simulink model "TV_2017old"  (R2016a)
settings: Solver=FixedStepAuto  StartTime=0.0  StopTime=inf  FixedStep=0.001  RelTol=1e-3
PreLoadFcn:
  | TV_2017_parameters
values from neighbouring files (symbols this model uses):
  battery_voltage = single(530)    [HIL_parameters.m]    (also in HIL_parameters_2018.m; TV_2017_parameters.m; TV_2017_parameters_VD.m)
  car_params = Simulink_Car_params    [HIL_parameters.m]    (also in HIL_parameters_2018.m; TV_2017_parameters.m; TV_2017_parameters_VD.m)
  i_Diff = 16    [HIL_parameters.m]    (also in HIL_parameters_2018.m; TV_2017_parameters.m)
  Kp = 1    [HIL_parameters.m]    (also in HIL_parameters_2018.m; TV_2017_parameters.m; TV_2017_parameters_VD.m)
  motor_data = struct    [HIL_parameters.m]    (also in HIL_parameters_2018.m; TV_2017_parameters.m)
  powerLimitControl = Simulink_el    [HIL_parameters.m]    (also in HIL_parameters_2018.m; TV_2017_parameters.m; TV_2017_parameters_VD.m)
  settings = Simulink_Settings    [HIL_parameters.m]    (also in HIL_parameters_2018.m; TV_2017_parameters.m; TV_2017_parameters_VD.m)
  SpdC_BCC = 0    [HIL_parameters.m]    (also in HIL_parameters_2018.m; TV_2017_parameters.m; TV_2017_parameters_VD.m)
  Speed_Neg_sat = -21    [HIL_parameters.m]    (also in HIL_parameters_2018.m; TV_2017_parameters.m; TV_2017_parameters_VD.m)
  Speed_Pos_sat = 21    [HIL_parameters.m]    (also in HIL_parameters_2018.m; TV_2017_parameters.m; TV_2017_parameters_VD.m)
  SteeringAngleFL = [-23.80 -22.65 -21.50 -20.34 -19.18 -18.03 -16.86 -15.70 -14.53 -13.35 -12.18 -10.99 -9.80 -8.61 -7.40 -6.19 -4.97 -3.75 -2.51 -1.26 0 1.27 2.56 3.85 5.17 6.50 7.84 9.21 10.59 12.00 13.42 14.88 16.36 17.87 19.41 20.99 22.61 24.26 25.97 27.73 29.54]    [CarSetupAnalysis2018.m]    (also in HIL_parameters_2018.m; TV_2017_parameters.m; TV_2017_parameters_VD.m = [-24.129 -22.950 -21.772 -20.593 -19.413 -18.232 -17.050 -15)
  SteeringAngleFR = [-29.54 -27.73 -25.97 -24.26 -22.61 -20.99 -19.41 -17.87 -16.36 -14.88 -13.42 -12.00 -10.59 -9.21 -7.84 -6.50 -5.17 -3.85 -2.56 -1.27 0 1.26 2.51 3.75 4.97 6.19 7.40 8.61 9.80 10.99 12.18 13.35 14.53 15.70 16.86 18.03 19.18 20.34 21.50 22.65 23.80]    [CarSetupAnalysis2018.m]    (also in HIL_parameters_2018.m; TV_2017_parameters.m; TV_2017_parameters_VD.m = [-29.3050 -27.5340 -25.8140 -24.1410 -22.5110 -20.9180 -19.3)
  SteeringWhAngle = [-105 -99.75 -94.5 -89.25 -84 -78.75 -73.5 -68.25 -63 -57.75 -52.5 -47.25 -42 -36.75 -31.5 -26.25 -21.0 -15.75 -10.5 -5.25 0.0 5.25 10.50 15.75 21.00 26.25 31.50 36.75 42.00 47.25 52.50 57.75  63.00 68.25 73.50 78.75 84.00 89.25 94.50 99.75 105.00]    [TV_2017_parameters_VD.m]
  Tn_n = 0    [HIL_parameters.m]    (also in HIL_parameters_2018.m; TV_2017_parameters.m; TV_2017_parameters_VD.m)
  tractionControl = Simulink_tc    [HIL_parameters.m]    (also in HIL_parameters_2018.m; IterativeTractionControlTuning.m; TV_2017_parameters.m; TV_2017_parameters_VD.m)
  yawRateControl = Simulink_yawRate    [HIL_parameters.m]    (also in HIL_parameters_2018.m; TV_2017_parameters.m; TV_2017_parameters_VD.m)
undefined symbols (not defined in the file or in its folder): DiscIntNeverNeededParam, magnitude, speedEstimation, TC_Decr_Gas, TC_Derivative, TC_Incr_Gas, TC_On, TC_Relay_Off, TC_Relay_On
libraries: CarMaker4SL x274, simulink_extras x45, simulink x37, dspfdesign x2
(part 9 of 14)

== matlab function TV_2017old/CarMaker/Control_System /Torque allocation 2016/Torque Allocation/TorqueAllocation ==
  data: Ti_lim output Bus: Ti_lim; T_req input; states input; maxMotorTorque input; settings parameter; car_params parameter; Mz_ref input; Ti_max output; Mz_error output; Mz_allocated output; yawRateControl parameter
function [Ti_lim,Ti_max,Mz_error, Mz_allocated]  = torqueAllocation(T_req,states,maxMotorTorque,settings, car_params, Mz_ref,yawRateControl)
%#codegen

%STATES
r = states.r;
negative_torque_limit = yawRateControl.negative_torque_limit;

%PARAMETERS
%mu = states.mu;
mu = settings.mu;
tf = car_params.t_f*2;
tr = car_params.t_r*2;
GR = car_params.GR;
r_eff = car_params.r_eff;
R = [r_eff; r_eff; r_eff; r_eff]';


Fzi = [max(1,states.Fz_FL) max(1,states.Fz_FR) max(1,states.Fz_RL) max(1,states.Fz_RR)]';
switch settings.TV_Method
    case 1
        % Only positive Torque
       alfa_r =  (Fzi(3) + Fzi(4)) / (Fzi(1) + Fzi(2) + Fzi(3) + Fzi(4));
    case 2
        % Can also allocate negative torque
       alfa_r =  (Fzi(3) + Fzi(4)) / (Fzi(1) + Fzi(2) + Fzi(3) + Fzi(4));
       %alfa_r = single(0.5)  test dette for å se om distribusjonen blir
       %lik ev soverestimer friksjonspotensialet
    case 3
        % Static 25 percent to each wheel
        alfa_r = single(0.5);
    case 4
        % Allocation with negative torque, but does not use Fz
        alfa_r = single(0.5); 
    otherwise
        alfa_r = single(0.5);       
end

S = states.wheel_angle;

l1 = car_params.t_f*cos(S);
l2 = car_params.t_f*cos(S);
l3 = car_params.t_r;
l4 = car_params.t_r;
L = [-l1; l2; -l3; l4];



%FIND MAXIMUM ALLOWED MOTOR TORQUE, TIRE/MOTOR
Ti_max          = single(zeros(4,1));
Ti_max_tire     = single(zeros(4,1));

RPM = [states.RPM_FL, states.RPM_FR, states.RPM_RL, states.RPM_RR];
Ti_max_motor = [maxMotorTorque.mmt_FL,maxMotorTorque.mmt_FR,maxMotorTorque.mmt_RL,maxMotorTorque.mmt_RR]; 

%Tire saturation based on mu and Fz
for i=1:4
    Ti_max_tire(i) = Fzi(i)*mu*R(i)/GR;
end

%Find minimum of tire saturation Torque and motor
for i=1:4
    Ti_max(i) = min(Ti_max_tire(i), Ti_max_motor(i));
end
%**********************************************%

T_F = single(zeros(2,1));
T_R = single(zeros(2,1));
sat_F = uint32(0);
sat_R = uint32(0);

if ( T_req >= 0)
    switch settings.TV_Method
        case 1
            % Only positive Torque
            [T_F, sat_F] = allocatePositiveTorque(Ti_max(1), Ti_max(2), T_req, R(1), R(2), (1-alfa_r), Mz_ref, GR, tf);
            [T_R, sat_R] = allocatePositiveTorque(Ti_max(3), Ti_max(4), T_req, R(3), R(4), alfa_r, Mz_ref, GR, tr);
        case 2
            % Can also allocate negative torque
            [T_F, sat_F] = allocateTorque(Ti_max(1), Ti_max(2), T_req, R(1), R(2), (1-alfa_r), Mz_ref, GR, tf, negative_torque_limit);
            [T_R, sat_R] = allocateTorque(Ti_max(3), Ti_max(4), T_req, R(3), R(4), alfa_r, Mz_ref, GR, tr ,negative_torque_limit);
        case 3
            % Static 25 percent to each wheel
            T_F = [0.25*T_req; 0.25*T_req];
            T_R = [0.25*T_req; 0.25*T_req];
        case 4
            % Allocation with negative torque, but does not use Fz
            [T_F, sat_F] = allocateTorque(Ti_max_motor(1), Ti_max_motor(2), T_req, R(1), R(2), (1-alfa_r), Mz_ref, GR, tf, negative_torque_limit);
            [T_R, sat_R] = allocateTorque(Ti_max_motor(3), Ti_max_motor(4), T_req, R(3), R(4), alfa_r, Mz_ref, GR, tr ,negative_torque_limit);
    end
            
    if ( (sat_F == 1) && (sat_R == 1) )
        % Nothing more to do
    elseif ( (sat_F == 1) && (sat_R == 0) )     
         if ( T_F(1) < 0) 
            T_remaining = T_req - (T_F(2));
         elseif (T_F(2) < 0) 
             T_remaining = T_req - (T_F(1));
         else
             T_remaining = T_req - (T_F(1) + T_F(2));
         end
         
         if (yawRateControl.enable == 1)
             Mz_remaining = Mz_ref - (-l1*GR*T_F(1)/R(1) + l2*GR*T_F(2)/R(2));
         else
             Mz_remaining = single(0);
         end 
         
        switch settings.TV_Method
            case 1
                % Only positive Torque
                [T_R sat_R] = allocatePositiveTorque(Ti_max(3), Ti_max(4), T_remaining, R(3), R(4), 1 , Mz_remaining, GR, tr);
            case 2
                % Can also allocate negative torque
                [T_R sat_R] = allocateTorque(Ti_max(3), Ti_max(4), T_remaining, R(3), R(4), 1 , Mz_remaining, GR, tr,negative_torque_limit);
            case 4
                [T_R sat_R] = allocateTorque(Ti_max_motor(3), Ti_max_motor(4), T_remaining, R(3), R(4), 1 , Mz_remaining, GR, tr,negative_torque_limit);
        end 
    elseif ( (sat_F == 0) && (sat_R == 1) )
         if ( T_R(1) < 0) 
            T_remaining = T_req - (T_R(2));
         elseif (T_R(2) < 0) 
             T_remaining = T_req - (T_R(1));
         else
             T_remaining = T_req - (T_R(1) + T_R(2));
         end        
        % For example rear is saturated, and front can still use more torque
        %T_remaining = T_req - (T_R(1) + T_R(2));
        if (yawRateControl.enable == 1)
             Mz_remaining = Mz_ref - (-l3*GR*T_R(1)/R(3) + l4*GR*T_R(2)/R(4));
        else
             Mz_remaining = single(0);
        end 
        %Mz_remaining = Mz_ref*(1-alfa_r);
        switch settings.TV_Method
            case 1
                % Only positive Torque
                 [T_F sat_F] = allocatePositiveTorque(Ti_max(1), Ti_max(2), T_remaining, R(1), R(2), 1 , Mz_remaining, GR, tf);
            case 2
                % Can also allocate negative torque
                [T_F sat_F] = allocateTorque(Ti_max(1), Ti_max(2), T_remaining, R(1), R(2), 1 , Mz_remaining, GR, tf,negative_torque_limit);
            case 4
                [T_F sat_F] = allocateTorque(Ti_max_motor(1), Ti_max_motor(2), T_remaining, R(1), R(2), 1 , Mz_remaining, GR, tf,negative_torque_limit);
        end      
    else
        %both false
        % Nothing to do here either
    end
else
    %REGENERATIVE BRAKE COMMAND ( T_DRIVER_REQ < 0 )
    switch settings.TV_Method
        case 1
            % Only positive Torque
            [T_F, sat_F] = allocateKersTorque(Ti_max(1), Ti_max(2), T_req, R(1), R(2), (1-alfa_r), Mz_ref, GR, tf);
            [T_R, sat_R] = allocateKersTorque(Ti_max(3), Ti_max(4), T_req, R(3), R(4), alfa_r, Mz_ref, GR, tr);
            
        case 2
            % Can also allocate negative torque
            [T_F, sat_F] = allocateKersTorque(Ti_max(1), Ti_max(2), T_req, R(1), R(2), (1-alfa_r), Mz_ref, GR, tf);
            [T_R, sat_R] = allocateKersTorque(Ti_max(3), Ti_max(4), T_req, R(3), R(4), alfa_r, Mz_ref, GR, tr);
        case 3
            % Static 25 percent to each wheel
            T_F = [0.25*T_req; 0.25*T_req];
            T_R = [0.25*T_req; 0.25*T_req];
        case 4
            % Allocation with negative torque, but does not use Fz
            [T_F, sat_F] = allocateKersTorque(Ti_max_motor(1), Ti_max_motor(2), T_req, R(1), R(2), (1-alfa_r), Mz_ref, GR, tf);
            [T_R, sat_R] = allocateKersTorque(Ti_max_motor(3), Ti_max_motor(4), T_req, R(3), R(4), alfa_r, Mz_ref, GR, tr);
    end
    if (sat_F == 1 && sat_R == 1)
        %Nothing more to do
        
    elseif (sat_F == 1 && sat_R == 0)
         T_remaining = T_req - (T_F(1) + T_F(2));
         %Disable Mz_remaining if yaw control disabled?
        if (yawRateControl.enable == 1)
             Mz_remaining = Mz_ref - (-l1*GR*T_F(1)/R(1) + l2*GR*T_F(2)/R(2));
        else
             Mz_remaining = single(0);
        end
        switch settings.TV_Method
            case 1
                % Only positive Torque
                [T_R sat_R] = allocateKersTorque(Ti_max(3), Ti_max(4), T_remaining, R(3), R(4), 1 , Mz_remaining, GR, tr);

            case 2
                % Can also allocate negative torque
                [T_R sat_R] = allocateKersTorque(Ti_max(3), Ti_max(4), T_remaining, R(3), R(4), 1 , Mz_remaining, GR, tr);
            case 3
                % Static 25 %
            case 4
                % Allocation with negative torque, but does not use Fz
                [T_R sat_R] = allocateKersTorque(Ti_max_motor(3), Ti_max_motor(4), T_remaining, R(3), R(4), 1 , Mz_remaining, GR, tr);
        end
        
    elseif (sat_F == 0 && sat_R == 1)
        %For example rear is saturated, and front can still use more torque
        T_remaining = T_req - (T_R(1) + T_R(2));
        %Mz_remaining = Mz_ref*(1-alfa_r);
        
        if (yawRateControl.enable == 1)
             Mz_remaining = Mz_ref - (-l3*GR*T_R(1)/R(3) + l4*GR*T_R(2)/R(4));
        else
             Mz_remaining = single(0);
        end
        switch settings.TV_Method
            case 1
                % Only positive Torque
                [T_F sat_F] = allocateKersTorque(Ti_max(1), Ti_max(2), T_remaining, R(1), R(2), 1 , Mz_remaining, GR, tf); 

            case 2
                % Can also allocate negative torque
                [T_F sat_F] = allocateKersTorque(Ti_max(1), Ti_max(2), T_remaining, R(1), R(2), 1 , Mz_remaining, GR, tf); 
            case 3
                % Static 25 %
            case 4
                % Allocation with negative torque, but does not use Fz
                [T_F sat_F] = allocateKersTorque(Ti_max_motor(1), Ti_max_motor(2), T_remaining, R(1), R(2), 1 , Mz_remaining, GR, tf);             
        end
    else
        %both false
        %Nothing to do here either
    end
end

Ti_all = [T_F' T_R'];

Ti_lim_struct = struct;
Ti_lim_struct.FL = Ti_all(1);
Ti_lim_struct.FR = Ti_all(2);
Ti_lim_struct.RL = Ti_all(3);
Ti_lim_struct.RR = Ti_all(4);

Ti_lim = Ti_lim_struct;

% Calculate what yaw moment that was achieved with the current 
% allocation
Fx_all = prod([Ti_all; 1./R;])*GR;
Mz_allocated = L'*Fx_all';
Mz_error = Mz_ref - Mz_allocated;
end


function [T, sat] = allocateTorque(L_max, R_max, T_req,...
          R_eff_L, R_eff_R, alfa, Mz_ref, GR, t, negative_torque_limit)
      
    T = single(zeros(2,1));
    sat = uint32(0);
    % Desired torque vectoring torque
    TV_des = abs(alfa*Mz_ref*R_eff_L/(GR*t)) + abs(alfa*Mz_ref*R_eff_R/(GR*t));
    % Take absolute value since T_req can be negative in case of KERS
    T_driver = alfa*T_req;

    if ( Mz_ref <= 0)
        % Implies that left side should realize the TV torque,
        % since only torque >= 0 is used here.
        % Mz is defined positive counter clockwise
        L = min( [TV_des, T_driver, L_max]); 
        if ( (L < TV_des) ) %&& (T_driver > 0))
            % Not fulfilled desired yaw moment
            R = - min( [(TV_des - L), R_max, negative_torque_limit]);
            T = [L;R];
        else
            max_t_add = min([(L_max-TV_des), R_max, (T_driver-L)/2]);
            L = L + max_t_add;
            R = max_t_add;
            T = [L;R];
        end
        % Floats comparison
        if ( (L + 0.001) < (T_driver))
            sat = uint32(1);
        end
        return;
    else
        R = min( [TV_des, T_driver, R_max]);
        %Max torque that can be added to both  
        if ( (R < TV_des) ) % && (T_driver > 0) )
            L = -min( [(TV_des - R), L_max,negative_torque_limit]);
            T = [L;R];
        else
            max_t_add = min([(R_max - TV_des),L_max, (T_driver-R)/2]);
            R = R + max_t_add;
            L = max_t_add;
            T = [L;R];
        end
        
        if ( (R + 0.001) < (T_driver))
            sat = uint32(1);
        end
        return;
    end
end

function [T, sat] = allocateKersTorque(L_max, R_max, T_req, R_eff_L, R_eff_R, alfa, Mz_ref, GR, t )
    T = single(zeros(2,1));
    sat = uint32(0);
    % Desired torque vectoring torque
    TV_des = abs(alfa*Mz_ref*R_eff_L/(GR*t)) + abs(alfa*Mz_ref*R_eff_R/(GR*t));
    % Take absolute value since T_req can be negative in case of KERS
    T_driver = abs(alfa*T_req);
   
    if (Mz_ref + 0.0001 >= 0)
        % Positive Mz_ref requires left side (inner wheels)
        % to brake more than the outer wheels.
        L = min( [TV_des, T_driver, L_max]);
        %Max torque that can be added to both
        if L_max < abs(TV_des)
            max_t_add = single(0);
        else
            max_t_add = min([(L_max-TV_des), R_max, (T_driver-L)/2]);
        end 
        L = - (L + max_t_add);
        R = - max_t_add;
        T = [L;R];
        % Floats comparison
        if ( (abs(L) + abs(R) + 0.001) < T_driver)
            sat = uint32(1);
        end
        return;
    else
        R = min( [abs(TV_des), T_driver, R_max]);
        %Max torque that can be added to both
        if R_max < abs(TV_des)
            max_t_add = single(0);
        else
            max_t_add = min([(R_max-abs(TV_des)), L_max, (T_driver-R)/2]);
        end
        R = - (R + max_t_add);
        L = - max_t_add;
        T = [L;R];
        % Floats comparison
        if ( (abs(L) + abs(R) + 0.001) < T_driver)
            sat = uint32(1);
        end
        return;
    end
end
function [T, sat] = allocatePositiveTorque(L_max, R_max, T_req,...
          R_eff_L, R_eff_R, alfa, Mz_ref, GR, t )
      
    T = single(zeros(2,1));
    sat = uint32(0);
    % Desired torque vectoring torque
    TV_des = abs(alfa*Mz_ref*R_eff_L/(GR*t)) + abs(alfa*Mz_ref*R_eff_R/(GR*t));
    % Take absolute value since T_req can be negative in case of KERS
    T_driver = alfa*T_req;

    if ( Mz_ref <= 0)
        % Implies that left side should realize the TV torque,
        % since only torque >= 0 is used here.
        % Mz is defined positive counter clockwise
        L = min( [TV_des, T_driver, L_max]);
        %Max torque that can be added to both
        %Skal det ikke være L < TV_des
        if L_max < abs(TV_des)
            max_t_add = single(0);
        else
            max_t_add = min([(L_max-TV_des), R_max, (T_driver-L)/2]);
        end 
        L = L + max_t_add;
        R = max_t_add;
        T = [L;R];  
        % Floats comparison
        if ( (L + R + 0.001) < (T_driver))
            sat = uint32(1);
        end
        return;
    else
        R = min( [abs(TV_des), T_driver, R_max]);
        %Max torque that can be added to both
        if R_max < abs(TV_des)
            max_t_add = single(0);
        else
            max_t_add = min([(R_max-abs(TV_des)),L_max, (T_driver-R)/2]);
        end
        R = R + max_t_add;
        L = max_t_add;
        T = [L;R];
        % Floats comparison
        if ( (L + R + 0.001) < (T_driver))
            sat = uint32(1);
        end
        return;
    end
end

== matlab function TV_2017old/CarMaker/Estimations/1st_deriv/Diff_Function ==
  data: y_old output; y_old input; sensors input; y output; delta_t input; RPM_der output
function [y_old,y , RPM_der] = innerFunction(y_old, sensors, delta_t)

y_old = single(circshift(y_old,1));
y_old(1) = sensors.RPM_FL;
        
RPM_der = single(sensors.RPM_der_FL);

M = length(y_old);
N = 3;
nu = 1;
j = 1;

k = 1:M;

x = phi(M,N,nu,j,k,delta_t) .* y_old;

y = single(sum(x));

end

function p = phi(M,N,nu,j,k,delta_t)

fac = (factorial(N + j + nu + 1) .*...
    factorial(N + 1)) ./...
    (M .* delta_t) .^ j;

[i,k2,k1,k] = ndgrid(0:nu + N,0:j,0:N-j,k);

eliminator = i > nu + k1 + k2;

evalIn = inPhi(M,N,nu,j,k,i,k1,k2);
evalIn(eliminator) = 0;

p = fac * sum(sum(sum(evalIn)));

p = p(:);

end

function p = inPhi(M,N,nu,j,k,i,k1,k2)

p = ((-1).^(N + i - k1 - k2) .*...
    ((k./M).^(N + i - k1 - k2 + 1) - ...
    ((k-1)./M).^(N + i - k1 - k2 + 1)))./...
    (factorial(k1) .* factorial(k2) .* factorial(i).*...
    factorial(N - j - k1) .*...
    factorial(j - k2) .*...
    factorial(N - k1 - k2) .*...
    factorial(nu - i + k1 + k2) .*...
    (N - k1 + 1) .*...
    (N + i -k1 - k2 + 1));

end

function n = factorial(n)

fac = [1;1;2;6;24;120;720;5040;40320;362880;3628800;39916800;479001600;6227020800.00000;87178291200.0000;1307674368000.00;20922789888000.0;355687428096000;6.40237370572800e+15;1.21645100408832e+17;2.43290200817664e+18;5.10909421717094e+19;1.12400072777761e+21;2.58520167388850e+22;6.20448401733239e+23;1.55112100433310e+25;4.03291461126606e+26;1.08888694504184e+28;3.04888344611714e+29;8.84176199373970e+30;2.65252859812191e+32;8.22283865417792e+33;2.63130836933694e+35;8.68331761881189e+36;2.95232799039604e+38;1.03331479663861e+40;3.71993326789901e+41;1.37637530912263e+43;5.23022617466601e+44;2.03978820811974e+46;8.15915283247898e+47;3.34525266131638e+49;1.40500611775288e+51;6.04152630633738e+52;2.65827157478845e+54;1.19622220865480e+56;5.50262215981209e+57;2.58623241511168e+59;1.24139155925361e+61;6.08281864034268e+62;3.04140932017134e+64];
n(n<0) = 0;
n = fac(n + 1);

end

== matlab function TV_2017old/CarMaker/Debug Information /Vehicle dynamics analysis JMH/MATLAB Function1 ==
  data: Force input; MM output; Moment input; car_params parameter
function MM = MagicMumber(Force,Moment,car_params)
WB = car_params.l;              % Wheelbase
Lf = 2.03-car_params.AeroRefX;  % Distance from aero referance to front axle
Fz = Force(3);                  % aerodynamic lift
PM = Moment(2);                 % aerodynamic pitch moment
Fr = (-PM-Fz.*Lf)./WB;           % aerodynamic load rear axle
Ff = -Fz-Fr;                    % aerodynamic load front axle
MM = Fr./(Ff+Fr);               % front-rear aerodynamic balance metric
end

== matlab function TV_2017old/CarMaker/Debug Information /Vehicle dynamics analysis JMH/MATLAB Function ==
  data: V input; OM_transient output; Delta input; Ay input; YawRate input; car_params parameter; OM_steadystate output
function [OM_transient,OM_steadystate] = OversteerMetric(V,Delta,Ay,YawRate,car_params)
W = car_params.l;
avgDelta = mean(Delta).*pi/180;     
AKR = V.*tan(avgDelta)./W;
OM_transient = YawRate-AKR;
OM_steadystate = (Ay.*W)./V.^2-avgDelta;
end

== matlab function TV_2017old/CarMaker/Control_System /Power Limit Torque Reduction Controller /Powerlimiting_Control_block ==
  data: states input; Motor_Efficiencies input; FL output; Ti_lim input; FR output; RL output; RR output; state output; powerLimitControl parameter; test1 output; test2 output; test3 output; test4 output
function [FL, FR, RL, RR,state,test1, test2,test3,test4 ] = Powerlimiting(states,Motor_Efficiencies,Ti_lim,powerLimitControl)
%#codegen
c = single(2*pi/60);

%% calculating wanted mechanical power
P_m_FL = states.RPM_FL*Ti_lim.FL*c;
P_m_FR = states.RPM_FR*Ti_lim.FR*c;
P_m_RR = states.RPM_RR*Ti_lim.RR*c;
P_m_RL = states.RPM_RL*Ti_lim.RL*c;
%P_m_TOT = P_m_FL + P_m_FR + P_m_RL + P_m_RR; 
test1 = single(0);
test2 = single(0);
test3 = single(0);
test4 = single(0);

 %%
% P_m_FL = states.RPM_FL*Teststates.T_FL*c;
% P_m_FR = states.RPM_FR*Teststates.T_FR*c;
% P_m_RR = states.RPM_RR*Teststates.T_RR*c;
% P_m_RL = states.RPM_RL*Teststates.T_RL*c;
%totpow = P_m_FL;
   %Calculating electrical power

if powerLimitControl.enable ~= 1 %If state != 2, then this powerlimiting module is off
    FL = Ti_lim.FL;
    FR = Ti_lim.FR;
    RR = Ti_lim.RR;
    RL = Ti_lim.RL;
    state = single(10);
    test1 = state;
    
elseif (states.power>0)
    P_e_FL = P_m_FL/Motor_Efficiencies.Efficiency_FL;
    P_e_FR = P_m_FR/Motor_Efficiencies.Efficiency_FR;
    P_e_RR = P_m_RR/Motor_Efficiencies.Efficiency_RR;
    P_e_RL = P_m_RL/Motor_Efficiencies.Efficiency_RL;
    P_e_TOT = P_e_FL +P_e_FR +P_e_RR +P_e_RL;
    %totpow = single(1);
    
    

    state = P_e_TOT;
    
    if P_e_TOT>powerLimitControl.positive_power_limit            %Positive powerlimiting
        %Total error 
        error = powerLimitControl.p_positive*(P_e_TOT - powerLimitControl.positive_power_limit);
        %Individual power error
        error_FL_m = error*Motor_Efficiencies.Efficiency_FL/4;
        error_FR_m = error*Motor_Efficiencies.Efficiency_FR/4;
        error_RR_m = error*Motor_Efficiencies.Efficiency_RR/4;
        error_RL_m = error*Motor_Efficiencies.Efficiency_RL/4;
        %Resulting torque reduction 
        T_red_FL = error_FL_m / states.RPM_FL;
        T_red_FR = error_FR_m / states.RPM_FR;
        T_red_RR = error_RR_m / states.RPM_RR;
        T_red_RL = error_RL_m / states.RPM_RL;
        %Subtraction and final output
        FL = Ti_lim.FL-T_red_FL;
        FR = Ti_lim.FR-T_red_FR;
        RR = Ti_lim.RR-T_red_RR;
        RL = Ti_lim.RL-T_red_RL;
        %state = single(1);
       % totpow = error;
    else %Below Powerlimiting max
        FL = Ti_lim.FL;
        FR = Ti_lim.FR;
        RR = Ti_lim.RR;
        RL = Ti_lim.RL;
        %state = single(2);
    end
else   %negative powerlimting                                
    P_e_FL = P_m_FL*Motor_Efficiencies.Efficiency_FL*-1;
    P_e_FR = P_m_FR*Motor_Efficiencies.Efficiency_FR*-1;
    P_e_RR = P_m_RR*Motor_Efficiencies.Efficiency_RR*-1;
    P_e_RL = P_m_RL*Motor_Efficiencies.Efficiency_RL*-1;
    P_e_TOT = P_e_FL +P_e_FR +P_e_RR +P_e_RL;
   
  
    if P_e_TOT>powerLimitControl.negative_power_limit    %Breaking negative limit
        
        
        %Total error 
        error = powerLimitControl.p_negative*(P_e_TOT - powerLimitControl.negative_power_limit);
        %Individual power error
        error_FL_m = error/Motor_Efficiencies.Efficiency_FL/4;
        error_FR_m = error/Motor_Efficiencies.Efficiency_FR/4;
        error_RR_m = error/Motor_Efficiencies.Efficiency_RR/4;
        error_RL_m = error/Motor_Efficiencies.Efficiency_RL/4;
        %Resulting torque reduction 
        T_red_FL = error_FL_m / states.RPM_FL;
        T_red_FR = error_FR_m / states.RPM_FR;
        T_red_RR = error_RR_m / states.RPM_RR;
        T_red_RL = error_RL_m / states.RPM_RL;
        %Subtraction and final output
        FL = Ti_lim.FL-T_red_FL;
        FR = Ti_lim.FR-T_red_FR;
        RR = Ti_lim.RR-T_red_RR;
        RL = Ti_lim.RL-T_red_RL;
        state = single(1);
        %totpow = error;
    else %Above negative constraint
        FL = Ti_lim.FL;
        FR = Ti_lim.FR;
        RR = Ti_lim.RR;
        RL = Ti_lim.RL;
        state = single(0);
    end
end


end

== matlab function TV_2017old/CarMaker/Debug Information /Fz_Estimation/FzEstDamper ==
  data: sensors input Bus: SensorInputs; Fz_damp_FL input; Fz_damp_FR input; Fz_damper_est output Bus: normalForces; Fz_damp_RL input; Fz_damp_RR input; car_params parameter; alfa_r output
function [Fz_damper_est, alfa_r] =  FzEstDamp(sensors, Fz_damp_FL, Fz_damp_FR, Fz_damp_RL, Fz_damp_RR, car_params)
%#codegen

Ks_front    = car_params.spring_constant_front;
Ks_rear     = car_params.spring_constant_rear;

 

preload_front = car_params.preload_front_mm;
preload_rear = car_params.preload_rear_mm;

unsprung = car_params.unsprung_mass_per_wheel_newton;

%esimate forces from spring and damper

Fz_damper_est.FL = Ks_front*sensors.damper_pos_FL + Fz_damp_FL;% 
Fz_damper_est.FR = Ks_front*sensors.damper_pos_FR + Fz_damp_FR;% 
Fz_damper_est.RL = Ks_rear*sensors.damper_pos_RL + Fz_damp_RL;% 
Fz_damper_est.RR = Ks_rear*sensors.damper_pos_RR + Fz_damp_RR;% 

alfa_r = (Fz_damper_est.RL + Fz_damper_est.RR) / (Fz_damper_est.FL + Fz_damper_est.FR + Fz_damper_est.RL + Fz_damper_est.RR);

%add unsprung mass to Fz estimate only when spring is loaded
add_unsprung_threshold = 10;
if (Fz_damper_est.FL>add_unsprung_threshold)
    Fz_damper_est.FL = Fz_damper_est.FL + unsprung; 
end
if (Fz_damper_est.FR>add_unsprung_threshold)
    Fz_damper_est.FR = Fz_damper_est.FR + unsprung; 
end
if (Fz_damper_est.RL>add_unsprung_threshold)
    Fz_damper_est.RL = Fz_damper_est.RL + unsprung; 
end
if (Fz_damper_est.RR>add_unsprung_threshold)
    Fz_damper_est.RR = Fz_damper_est.RR + unsprung; 
end


end

== matlab function TV_2017old/CarMaker/Debug Information /Fz_Estimation/FzEstDamper 2016 ==
  data: sensors input Bus: SensorInputs; Fz_damp_FL input; Fz_damp_FR input; Fz_damper_est output Bus: normalForces; Fz_damp_RL input; Fz_damp_RR input; car_params parameter; alfa_r output
function [Fz_damper_est, alfa_r] =  FzEstDamp(sensors, Fz_damp_FL, Fz_damp_FR, Fz_damp_RL, Fz_damp_RR, car_params)
%#codegen

Ks_front    = car_params.spring_constant_front;
Ks_rear     = car_params.spring_constant_rear;

MR_front    = car_params.motion_ratio_front;
MR_rear     = car_params.motion_ratio_rear;     

preload_front = car_params.preload_front_mm;
preload_rear = car_params.preload_rear_mm;

%unsprung = car_params.unsprung_mass_per_wheel_newton;
% 0 - 1 mm, Go from 0 to neutral Fz
FL_scaling = single(min(sensors.damper_pos_FL, single(1)));
FR_scaling = single(min(sensors.damper_pos_FR, single(1)));
RL_scaling = single(min(sensors.damper_pos_RL, single(1)));
RR_scaling = single(min(sensors.damper_pos_RR, single(1)));

% Fz_damper_est.FL = (Ks_front*(sensors.damper_pos_FL + preload_front) + Fz_damp_FL)*MR_front + unsprung;
% Fz_damper_est.FR = (Ks_front*(sensors.damper_pos_FR + preload_front) + Fz_damp_FR)*MR_front + unsprung;
% Fz_damper_est.RL = (Ks_rear*(sensors.damper_pos_RL  + preload_rear)  + Fz_damp_RL)*MR_rear  + unsprung;
% Fz_damper_est.RR = (Ks_rear*(sensors.damper_pos_RR  + preload_rear)  + Fz_damp_RR)*MR_rear  + unsprung;

Fz_damper_est.FL = Ks_front*sensors.damper_pos_FL + Fz_damp_FL + (preload_front*Ks_front)*FL_scaling;
Fz_damper_est.FR = Ks_front*sensors.damper_pos_FR + Fz_damp_FR + (preload_front*Ks_front)*FR_scaling;
Fz_damper_est.RL = Ks_rear*sensors.damper_pos_RL + Fz_damp_RL + (preload_rear*Ks_rear)*RL_scaling;
Fz_damper_est.RR = Ks_rear*sensors.damper_pos_RR + Fz_damp_RR + (preload_rear*Ks_rear)*RR_scaling;

alfa_r = (Fz_damper_est.RL + Fz_damper_est.RR) / (Fz_damper_est.FL + Fz_damper_est.FR + Fz_damper_est.RL + Fz_damper_est.RR);
end

== matlab function TV_2017old/CarMaker/Debug Information /Fz_Estimation/FzEstLoadTransfer ==
  data: Fz_loadTransfer_est output Bus: normalForces; sensor input Bus: SensorInputs; car_params parameter; vx input
function Fz_loadTransfer_est  = FzEstLoadTransfer(sensor,car_params,vx)
%#codegen




mv = car_params.car_mass + car_params.driver_mass; % Total mass( driver + car) X
l  = car_params.l; %Wheel base X
lr = car_params.l_r; % X
lf = car_params.l_f;% X

ef = car_params.t_f*2; % Front track X
er = car_params.t_r*2; % Rear track X


hc = car_params.CoG_height; % X
g = 9.81; % X
air_density = single(1.2);

Fz_loadTransfer_est.FL = single(0);%(0.5*mv*(lr*g/l - hc*sensor.ax/l) - mv*(lr*g/l - hc*sensor.ax/l)*hc*sensor.ay/(ef*g))  + (vx^2 * car_params.aero_ref_area* car_params.aero_lift_coeff*air_density)/8;
Fz_loadTransfer_est.FR = single(0);%(0.5*mv*(lr*g/l - hc*sensor.ax/l) + mv*(lr*g/l - hc*sensor.ax/l)*hc*sensor.ay/(ef*g))  + (vx^2 * car_params.aero_ref_area* car_params.aero_lift_coeff*air_density)/8;
Fz_loadTransfer_est.RL = single(0);%(0.5*mv*(lf*g/l + hc*sensor.ax/l) - mv*(lf*g/l + hc*sensor.ax/l)*hc*sensor.ay/(er*g))  + (vx^2 * car_params.aero_ref_area* car_params.aero_lift_coeff*air_density)/8;
Fz_loadTransfer_est.RR = single(0);%(0.5*mv*(lf*g/l + hc*sensor.ax/l) + mv*(lf*g/l + hc*sensor.ax/l)*hc*sensor.ay/(er*g))  + (vx^2 * car_params.aero_ref_area* car_params.aero_lift_coeff*air_density)/8;

end

== matlab function TV_2017old/CarMaker/Debug Information /Subsystem/MATLAB Function ==
  data: RPM_FL_IN input; RPM_FR_IN input; RPM_RL_IN input; RPM_RR_IN input; Pm_FL output; T input; T_FL output; RPM_FL output; Pm_FR output; T_FR output; RPM_FR output; Pm_RL output; T_RL output; RPM_RL output; Pm_RR output; T_RR output; RPM_RR output
function [Pm_FL, T_FL, RPM_FL,Pm_FR, T_FR, RPM_FR,Pm_RL, T_RL,...
          RPM_RL,Pm_RR, T_RR, RPM_RR] = powerMeasurement(RPM_FL_IN, RPM_FR_IN,RPM_RL_IN,RPM_RR_IN, T)
%#codegen

%Conversion from RPM to rad/s
c = single(2*pi/60);

T_FL = T.FL;
T_FR = T.FR;
T_RL = T.RL;
T_RR = T.RR;

RPM_FL = RPM_FL_IN;
RPM_FR = RPM_FR_IN;
RPM_RL = RPM_RL_IN;
RPM_RR = RPM_RR_IN;


Pm_FL = RPM_FL*c*T.FL;
Pm_FR = RPM_FR*c*T.FR;
Pm_RL = RPM_RL*c*T.RL;
Pm_RR = RPM_RR*c*T.RR;

== matlab function TV_2017old/CarMaker/Control_System /Torque allocation 2017/Motor temperature limiter ==
  data: states input; maxMotorTorque output Bus: maxMotorTorque; settings parameter; car_params parameter
function maxMotorTorque = maxMotorTorque_MotorTemp(states,settings, car_params)
%#codegen

% The inverters limits output torque based on internal temperature
mmt = single(settings.max_motor_torque);
upper_max_temp = single(car_params.AMK_motor_upper_max_temp);
cutoff_temp    = single(car_params.AMK_motor_cutoff_temp);
torque = [mmt mmt 0]; %breakpoints for lookup function
temp = [0 upper_max_temp cutoff_temp];


mot_FL_temp = single(states.AMK_inverter_temp_FL);
mot_FR_temp = single(states.AMK_inverter_temp_RL);
mot_RL_temp = single(states.AMK_inverter_temp_RL);
mot_RR_temp = single(states.AMK_inverter_temp_RR);

%  y = interp1(xdata,ydata,x)
maxMotorTorque.mmt_FL = interp1(temp,torque,  mot_FL_temp  );
maxMotorTorque.mmt_FR = interp1(temp,torque,  mot_FR_temp  );
maxMotorTorque.mmt_RL = interp1(temp,torque,  mot_RL_temp  );
maxMotorTorque.mmt_RR = interp1(temp,torque,  mot_RR_temp  );

== matlab function TV_2017old/CarMaker/Control_System /2016 adapted/MATLAB Function ==
  data: states input; maxMotorTorque output Bus: maxMotorTorque; settings parameter
function maxMotorTorque = findMaxMotorTorque(states,settings)
%#codegen

% DC Voltage                             / states
% Max allowable current draw in total    /settings
% Load distribution                      /states

Fzi = [max(1,states.Fz_FL) max(1,states.Fz_FR) max(1,states.Fz_RL) max(1,states.Fz_RR)]';

switch settings.TV_Method
    case 1 % No negative torque
        alfa_r =  (Fzi(3) + Fzi(4)) / (Fzi(1) + Fzi(2) + Fzi(3) + Fzi(4));
    case 2 % with negative torque
        alfa_r =  (Fzi(3) + Fzi(4)) / (Fzi(1) + Fzi(2) + Fzi(3) + Fzi(4));
    case 3 % static 25 %
        alfa_r = single(0.5);
    case 4 % with negative torque, no Fz
        alfa_r = single(0.5);
    otherwise
        alfa_r = single(0.5);
end

RPM_to_angular = single(2*pi/60);
omega_FL = states.RPM_FL*RPM_to_angular;
omega_FR = states.RPM_FR*RPM_to_angular;
omega_RL = states.RPM_RL*RPM_to_angular;
omega_RR = states.RPM_RR*RPM_to_angular;

mmt = settings.max_motor_torque;
available_power = states.DC_voltage*settings.max_battery_discharge;

max_torque_front = min(mmt, (available_power*(1-alfa_r))/ (2 * max( max(1,omega_FL), max(1,omega_FR))) );
max_torque_rear = min(mmt, (available_power*alfa_r)     / (2 * max( max(1,omega_RL), max(1,omega_RR))) );
                      
maxMotorTorque.mmt_FL = max_torque_front;
maxMotorTorque.mmt_FR = max_torque_front;
maxMotorTorque.mmt_RL = max_torque_rear;
maxMotorTorque.mmt_RR = max_torque_rear;

== matlab function TV_2017old/CarMaker/Control_System /Torque allocation 2017/Torque Allocation Quadratic Programming ==
  data: Mz_ref input; Ti_lim output Bus: Ti_lim; T_req input; states input; maxMotorTorque input; settings parameter; car_params parameter; yawRateControl parameter; saturated_constraints output; powerLimitControl parameter
function [Ti_lim, saturated_constraints] = QP(Mz_ref, T_req, states, maxMotorTorque, settings, car_params, yawRateControl, powerLimitControl)


max_matrix_dimention = 17;
Ti_max = [0 0 0 0];
Mz_allocated = single(0);
saturated_constraints = [0 0 0 0];
% ------- STATES -------------
r = states.r;
negative_torque_limit = yawRateControl.negative_torque_limit;

%---------- PARAMETERS -------
TV_method = settings.TV_Method;
mmt = single(settings.max_motor_torque);
mu = settings.mu;
lf = car_params.l_f;
lr = car_params.l_r;
tf = car_params.t_f;
tr = car_params.t_r;
arm_f = sqrt(tf^2 + lf^2);
GR = car_params.GR;
r_eff = car_params.r_eff;
R = [r_eff, r_eff, r_eff, r_eff]; % todo -> account for load
delta = states.wheel_angle;
delta_FL = delta;   % fix for later  ->individual steer angles
delta_FR = delta;
T_abs = abs(T_req); 
Mz_ref_scaled = Mz_ref * single(yawRateControl.enable);
pow_lim         = powerLimitControl.positive_power_limit; %= single(75000); % Positive effect limit
neg_pow_lim     = powerLimitControl.negative_power_limit;
error = 0;

rads_FL = max(10,abs(states.RPM_FL))*2*pi/60  *sign(states.RPM_FL);
rads_FR = max(10,abs(states.RPM_FR))*2*pi/60  *sign(states.RPM_FL);
rads_RL = max(10,abs(states.RPM_RL))*2*pi/60  *sign(states.RPM_FL);
rads_RR = max(10,abs(states.RPM_RR))*2*pi/60  *sign(states.RPM_FL);

mmt_FL = min(mmt, max(0.1, maxMotorTorque.mmt_FL));  % fix ned limit later
mmt_FR = min(mmt, max(0.1, maxMotorTorque.mmt_FR)); 
mmt_RL = min(mmt, max(0.1, maxMotorTorque.mmt_RL)); 
mmt_RR = min(mmt, max(0.1, maxMotorTorque.mmt_RR)); 
minmt_FL = min([mmt_FL settings.max_motor_brake_torque]);
minmt_FR = min([mmt_FR settings.max_motor_brake_torque]);
minmt_RL = min([mmt_RL settings.max_motor_brake_torque]);
minmt_RR = min([mmt_RR settings.max_motor_brake_torque]);
%***************************************************

M_T_FL =     GR/R(1) *  -sin(  atan(tf/lf)  -  delta_FL)  *arm_f;
M_T_FR =     GR/R(2) *   sin(  atan(tf/lf)  +  delta_FR)  *arm_f;
M_T_RL =     GR/R(3) *  -tr;
M_T_RR =     GR/R(4) *   tr;

%***************************************************

G_1       = 2*[ M_T_FL^2         ,          M_T_FL *M_T_FR   ,       M_T_FL*M_T_RL   ,        M_T_FL*M_T_RR    ;
               M_T_FR * M_T_FL    ,           M_T_FR^2        ,       M_T_FR*M_T_RL   ,        M_T_FR*M_T_RR    ;
               M_T_RL * M_T_FL    ,        M_T_RL*M_T_FR      ,         M_T_RL^2      ,        M_T_RL*M_T_RR    ;
               M_T_RR * M_T_FL    ,        M_T_RR*M_T_FR      ,      M_T_RR* M_T_RL   ,            M_T_RR^2  ];

G_2  =[        2/mmt_FL^2,    0,          0,          0;
                  0,      2/mmt_FR^2,     0,          0;
                  0,          0,      2/mmt_RL^2,     0;
                  0,          0,          0,      2/mmt_RR^2];
              
G_3 =[
    ];

G = G_1/100 + 100000*G_2;

c       = [M_T_FL  , M_T_FR  , M_T_RL  ,  M_T_RR    ]'*-2*Mz_ref_scaled;      

A_eq   =  single([ 1   1   1   1 ]);
b_eq   =  T_req ;

A      =     single([rads_FL ,   rads_FR ,   rads_RL ,    rads_RR   ;
                         1    ,       0    ,       0    ,        0      ;
                         0    ,       1    ,       0    ,        0      ;
                         0    ,       0    ,       1    ,        0      ;
                         0    ,       0    ,       0    ,        1      ;
                        -1    ,       0    ,       0    ,        0      ;
                         0    ,      -1    ,       0    ,        0      ;
                         0    ,       0    ,      -1    ,        0      ;
                         0    ,       0    ,       0    ,       -1      ]);

b    =  [pow_lim ,  mmt_FL  ,    mmt_FR  ,    mmt_RL  ,     mmt_RR    , mmt_FL  ,  mmt_FR  ,  mmt_RL  ,   mmt_RR ]'; 
% ------------------- POWLIM not done !! is done for now? compensate for efficiency later?`-------------------
%Determine feasible startingpoint  / scale problem
%function [b_eq, x_o]  = determine_feasible_startingpoint(A,b,b_eq,pow_lim,T)

if b_eq > 0
    beta = b_eq /(-b(2) -b(3) -b(4) -b(5));
elseif b_eq < 0 
    beta = b_eq /(-b(6) -b(7) -b(8) -b(9)); 
else
    beta = single(0);
end


if (beta < 1)&&(beta > 0.001) % a feasible startingpoint exists (considering b(2:end))
    x_0 = beta * [-b(2) -b(3) -b(4)  -b(5)]';
    pow = -A(1,:)*x_0;
    if pow>pow_lim
        b_eq = T_req * (pow_lim/pow);
        x_0 = x_0*(pow_lim/pow);
    end
    x = active_set(G,c,A,b,A_eq,b_eq,x_0);
   
elseif (beta > -1)&&(beta < -0.001) % a feasible startingpoint exists (considering b(2:end))
    x_0 = beta * [-b(6) -b(7) -b(8)  -b(9)]';
    pow = -A(1,:)*x_0;
    if pow>pow_lim
        b_eq = T_req * (pow_lim/pow);
        x_0 = x_0*(pow_lim/pow);
    end
    x = active_set(G,c,A,b,A_eq,b_eq,x_0);
   
   
elseif (beta >= 1) % a feasible startingpoint does not exist (considering b(2:end))
    x_0 = [ -b(2)   -b(3) -b(4)  -b(5)]'; 
    pow = -A(1,:)*x_0;
    if pow>pow_lim
        b_eq = T_req * (pow_lim/pow);
        x_0 = x_0*(pow_lim/pow);
    end
    x = x_0;
else
    x = zeros(4,1,'single'); %default case, should not happen
end




% add constraints active based on lambda
Mz_allocated = [M_T_FL  , M_T_FR  , M_T_RL  ,  M_T_RR  ]* x;
Ti_lim_struct    = struct;
Ti_lim_struct.FL = x(1); Ti_lim_struct.FR = x(2); Ti_lim_struct.RL = x(3); Ti_lim_struct.RR = x(4);
Ti_lim = Ti_lim_struct;
active_const = [0 0 0 0];
end

%Active set method for convex QP  ( pg 472 optreg ) 
function x = active_set(G,c,A,b,A_eq,b_eq,x_0)

%0) Formulate KKT matrix

%1) set w_0 to be a subset of the actiive constraints at x_o


W_i = zeros(1,size(A,1),'single'); % W_i lists indexes of A in W
x_k = x_0;
x = single(x_0);


debug_main_iteration = 1;
notdone = 1;
iteration_count = 0;

while notdone
    if iteration_count > 100;
        disp('iteration-count overflow!')
        notdone = 0;
        x = x_k;
    end
    
   
    [p_k, all_lambda_positive] = calc_p_and_eval_lambda(G,  c,  A,  b, A_eq,  b_eq, W_i,  x_k );
    
    
    %debug-----------------------------------------------------------
    
    [alpha,violating_indexes] = compute_alpha(A,b,x_k,p_k,W_i);
    de_bug2 = A*(x_k + alpha*p_k) - b;
    ansr = min(de_bug2);
    if ansr < -0.01
        fail = true;
    end
    
    [p_k, all_lambda_positive] = calc_p_and_eval_lambda(G,  c,  A,  b, A_eq,  b_eq, W_i,  x_k ); 
    %debug________________________________________________
    
    if sum(abs(p_k)) <= 0.01
        if all_lambda_positive; 
            x = x_k;
            notdone = 0;
           
        else
            W_i = exclude_most_negative_lambda_index(G,  c,  A,  b,  A_eq,  b_eq,  x_k , W_i);
            iteration_count = iteration_count + 1;
        end
    elseif sum(abs(p_k)) ~= 0
        [alpha,violating_indexes] = compute_alpha(A,b,x_k,p_k,W_i);
        x_k = x_k + alpha*p_k ;
        if alpha < 1 %indicates blocking constraints
%           disp('blocking constraints')
            disp(alpha)
            %add one of blocking constraints to W_k
            new_index = find(violating_indexes,1); %returns index of first non-0 value
            W_i(new_index) = 1;
            iteration_count = iteration_count + 1;
        else
             
            iteration_count = iteration_count + 1;
        end
    else
        
        x = x_k;
        iteration_count = 105;
    end
end

% make it based on lambda
end

function [p_val, all_lambda_positive] =  calc_p_and_eval_lambda(G,  c,  A,  b, A_eq,  b_eq, W_i, x_k )
[W,b_w] = construct_working_set(A,  b, A_eq , b_eq ,  W_i);    
[p, lagrangians] = solve_KKT(G,  c,  W,  b_w,  x_k );
p_val = p;
%all_lambda_positive = sum(sign(lagrangians)) == (sum(W_i)+1);% indicates all values are positivr ( sign(0) returns false, will this cause error on loosely active constraints?  edit:  yes it did ....

if length(lagrangians)==size(b_eq,1)
    all_lambda_positive = true;
else
    all_lambda_positive = min(lagrangians((length(b_eq)+1):end)) >= 0; % indicates all values are positive       
end
end

function W_i = exclude_most_negative_lambda_index(G,  c,  A,  b,  A_eq, b_eq,  x_k , W_i)
[W,b_w] = construct_working_set(A,  b, A_eq , b_eq , W_i);   
[~, lagrangians] = solve_KKT(G,  c,  W,  b_w,  x_k );
% identify most negative lagrangian / 1 negative is guarranteed to exist
            low_value = single(0);
            low_index = int8(1);
            for j = (length(b_eq)+1):length(lagrangians)
                if lagrangians(j) <= low_value
                    low_value = lagrangians(j);
                    low_index = int8(j-1);
                else
                    %skip
                end
            end
            k = find(W_i,low_index);
            if k(low_index) > length(W_i)
                r=9;
            end
            W_i(k(low_index)) = 0;
            %W_i(low_index) = 0; % exclude j from IandW
            % construct new working set
            %[W,b_w] = construct_working_set(A_eq, b_eq, A, W_i, b);
            % got out of range error, tried to access second nonzero
            % element in W_i when there only where one nonzero elemnt (pow lim )
end

function [p, lambda_s] = solve_KKT(G,  c,  A,  b,  x_k )  % A is the working set W 
    sol = zeros(4+size(A,1),1,'single');
    %   add error handling here? 
    %   G, A and K needs full rank for K to be invertable
    
    h =  A*x_k   -   b           ;
    g =  c       +   G*x_k       ;
    K = [G             A'        ;
         A        zeros(size(A,1),'single')];
    
    sol      =   K\[g ; h];
    p        =   -sol(1:size(G,1));
    lambda_s =    sol((size(G,1)+1):size(G,1)+size(A,1));
end
 
function [alpha,violating_indexes] = compute_alpha(A, b , x_k , p_k ,  W_i) %% this is wrong, observed alpha -368.3450
    
    violating_indexes = zeros(1,size(A,1));
    values = ones(1,size(A,1));
    debug_values = ones(1,size(A,1));
    for i =  1:size(A,1) 
        if ~W_i(i)  &&  (A(i,:)*p_k < 0)
            val = (b(i) - A(i,:)*x_k)/(A(i,:)*p_k);
            debug_values(i) = val;
            if 0<=val && val<=1
                values(i) = val;
                violating_indexes(i) = 1;
            end
        else
            %skip
        end
    end
    alpha = min([1,values]);
end

function [W,b_w] = construct_working_set(A , b, A_eq , b_eq  , W_i )
W_ineq = zeros( dim_bound(sum(W_i)) , dim_bound(size(A_eq,2)) , 'single' ); 
b_ineq = zeros( dim_bound(sum(W_i)) , 1 , 'single' );
working_set_iterator = 1;
for u=1:size(A,1)
        if W_i(u)==1
            
            W_ineq(working_set_iterator,:) = A(u,:);
            b_ineq(working_set_iterator,1) = b(u);
            working_set_iterator = working_set_iterator + 1;
        end
end
W = [A_eq ; W_ineq]; 
b_w = [b_eq;b_ineq];
end

function y = dim_bound(n)
assert (n <= 17);
y = n;
end

== matlab function TV_2017old/CarMaker/Control_System /Torque allocation 2017/max combined tire torque based on (Fz, SA,mu)  ==
  data: states input; maxMotorTorque output Bus: maxMotorTorque; settings parameter; car_params parameter; tractionControl parameter
function maxMotorTorque = maxTireForce(states,settings,car_params,tractionControl)
%#codegen
% draft scale function     (-x^4-x^2)/3 + -x^6/3  + 1
% calculate max tire force based on F_z and slip angle


% Need to be over a certain velocity for this to work....

v_x = states.V_x;
mu = settings.mu;
GR = car_params.GR;
r = car_params.r_eff;
max_slip = tractionControl.slip_ang_limit;
mmt = settings.max_motor_torque;

F_z_FL = states.Fz_FL;
F_z_FR = states.Fz_FR;
F_z_RL = states.Fz_RL;
F_z_RR = states.Fz_RR;

SA_norm_FL = states.SA_FL/max_slip;
SA_norm_FR = states.SA_FR/max_slip;
SA_norm_RL = states.SA_RL/max_slip;
SA_norm_RR = states.SA_RR/max_slip;

mu_scale_factor_FL = (-SA_norm_FL^4 -SA_norm_FL^2)/3 + -SA_norm_FL^6/3  + 1;
mu_scale_factor_FR = (-SA_norm_FR^4 -SA_norm_FR^2)/3 + -SA_norm_FR^6/3  + 1;
mu_scale_factor_RL = (-SA_norm_RL^4 -SA_norm_RL^2)/3 + -SA_norm_RL^6/3  + 1;
mu_scale_factor_RR = (-SA_norm_RR^4 -SA_norm_RR^2)/3 + -SA_norm_RR^6/3  + 1;

if v_x > 2;
    maxMotorTorque.mmt_FL = F_z_FL * mu_scale_factor_FL *mu * r/ GR ;
    maxMotorTorque.mmt_FR = F_z_FR * mu_scale_factor_FR *mu * r/ GR ;
    maxMotorTorque.mmt_RL = F_z_RL * mu_scale_factor_RL *mu * r/ GR ;
    maxMotorTorque.mmt_RR = F_z_RR * mu_scale_factor_RR *mu * r/ GR ;
else
    maxMotorTorque.mmt_FL = mmt;
    maxMotorTorque.mmt_FR = mmt;
    maxMotorTorque.mmt_RL = mmt;
    maxMotorTorque.mmt_RR = mmt;
end

end

== matlab function TV_2017old/CarMaker/Control_System /Torque allocation 2017/max long tire torque based on (FZ , mu) ==
  data: states input; maxMotorTorque output Bus: maxMotorTorque; settings parameter; car_params parameter
function maxMotorTorque = maxTireForce(states,settings, car_params)
%#codegen

% calculate max tire force based on F_z and slip angle
mu = settings.mu;
GR = car_params.GR;
r = car_params.r_eff;

F_z_FL = states.Fz_FL;
F_z_FR = states.Fz_FR;
F_z_RL = states.Fz_RL;
F_z_RR = states.Fz_RR;


maxMotorTorque.mmt_FL = F_z_FL * r * mu / GR ;
maxMotorTorque.mmt_FR = F_z_FR * r * mu / GR ;
maxMotorTorque.mmt_RL = F_z_RL * r * mu / GR ;
maxMotorTorque.mmt_RR = F_z_RR * r * mu / GR ;
